simulink model "proc_control_node"  (R2021b)
settings: Solver=FixedStepAuto  StartTime=0.0  StopTime=inf  FixedStep=simulink.sampletime  RelTol=1e-3
model workspace (MAT data in the model file):
  SL_ROS_VariableLengthArrays_MaxSizes.CommonInfo.ArrayTruncateAction = 'EmitWarning'
  SL_ROS_VariableLengthArrays_MaxSizes.MsgTypeMap = containers.Map
  SL_ROS_VariableLengthArrays_MaxSizes.MsgTypeMap.serialization.keys = {'trajectory_msgs/MultiDOFJointTrajectoryPoint'}
  SL_ROS_VariableLengthArrays_MaxSizes.MsgTypeMap.serialization.values{1}(1).PropertyName = 'Accelerations'
  SL_ROS_VariableLengthArrays_MaxSizes.MsgTypeMap.serialization.values{1}(1).DataType = 'geometry_msgs/Twist'
  SL_ROS_VariableLengthArrays_MaxSizes.MsgTypeMap.serialization.values{1}(1).MaxLength = 6000
  SL_ROS_VariableLengthArrays_MaxSizes.MsgTypeMap.serialization.values{1}(2).PropertyName = 'Transforms'
  SL_ROS_VariableLengthArrays_MaxSizes.MsgTypeMap.serialization.values{1}(2).DataType = 'geometry_msgs/Transform'
  SL_ROS_VariableLengthArrays_MaxSizes.MsgTypeMap.serialization.values{1}(2).MaxLength = 6000
  SL_ROS_VariableLengthArrays_MaxSizes.MsgTypeMap.serialization.values{1}(3).PropertyName = 'Velocities'
  SL_ROS_VariableLengthArrays_MaxSizes.MsgTypeMap.serialization.values{1}(3).DataType = 'geometry_msgs/Twist'
  SL_ROS_VariableLengthArrays_MaxSizes.MsgTypeMap.serialization.values{1}(3).MaxLength = 6000
  SL_ROS_VariableLengthArrays_MaxSizes.MsgTypeMap.serialization.uniformity = 0
  SL_ROS_VariableLengthArrays_MaxSizes.MsgTypeMap.serialization.keyType = 'char'
  SL_ROS_VariableLengthArrays_MaxSizes.MsgTypeMap.serialization.valueType = 'any'
undefined symbols (not defined in the file or in its folder): InitAUVPlant, InitController, MPC, physics, simulation, simulink
libraries: robotlib x36, aerolibutil x7, sharedtransform x5, simulink_extras x3
settings Model: SimulationMode=accelerator  PacingRate=1.400000  Creator=lamarre  LastModifiedBy=lamarre
settings OptimizationCC: StrengthReduction=on  PassReuseOutputArgsAs=Individual arguments  ZeroExternalMemoryAtStartup=off  ZeroInternalMemoryAtStartup=off  EfficientFloat2IntCast=on  LifeSpan=inf  MaxStackSize=64  OptimizeBlockOrder=speed  OptimizationPriority=Speed  MultiThreadedLoops=on  EfficientTunableParamExpr=on
settings DebuggingCC: ReadBeforeWriteMsg=DisableAll  WriteAfterWriteMsg=DisableAll  WriteAfterReadMsg=DisableAll  MultiTaskDSMMsg=none  ParameterTunabilityLossMsg=error  UnderSpecifiedDimensionMsg=warning
settings HardwareCC: ProdLargestAtomicInteger=Long  ProdLargestAtomicFloat=Double  ProdLongLongMode=on  ProdHWDeviceType=ARM Compatible->ARM 64-bit (LLP64)
settings ModelReferenceCC: UpdateModelReferenceTargets=IfOutOfDate
settings SFSimCC: SFSimEcho=off  MATLABDynamicMemAlloc=off  SimTargetLang=C++
settings RTWCC: Description=Embedded Coder  SystemTargetFile=ert.tlc  HardwareBoard=Robot Operating System (ROS)  TLCOptions="-aInlineSetEventsForThisBaseRateFcn=TLC_FALSE -aSuppressMultiTaskScheduler=TLC_FALSE  -aRateBasedStepFcn=0"  GenCodeOnly=on  TemplateMakefile=ert_default_tmf  Toolchain=Catkin  BuildConfiguration=Faster Runs  TargetLang=C++
settings CodeAppCC: ForceParamTrailComments=on  IgnoreCustomStorageClasses=off  IgnoreTestpoints=on  OperatorAnnotations=on  SimulinkDataObjDesc=on  SFDataObjDesc=on  InsertBlockDesc=on
settings ERTTargetCC: TargetLangStandard=C++11 (ISO)  CodeInterfacePackaging=C++ class  SupportContinuousTime=on  SupportVariableSizeSignals=on  ExtModeMexArgs='192.168.0.31' 0 17725  RootIOFormat=Structure reference

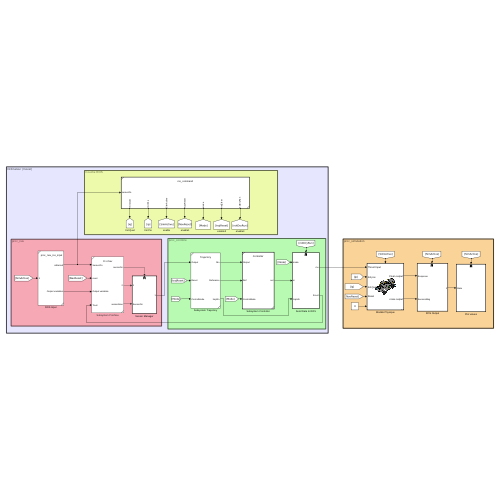
[thumbnail: Simulink's stored preview of the top-level diagram]
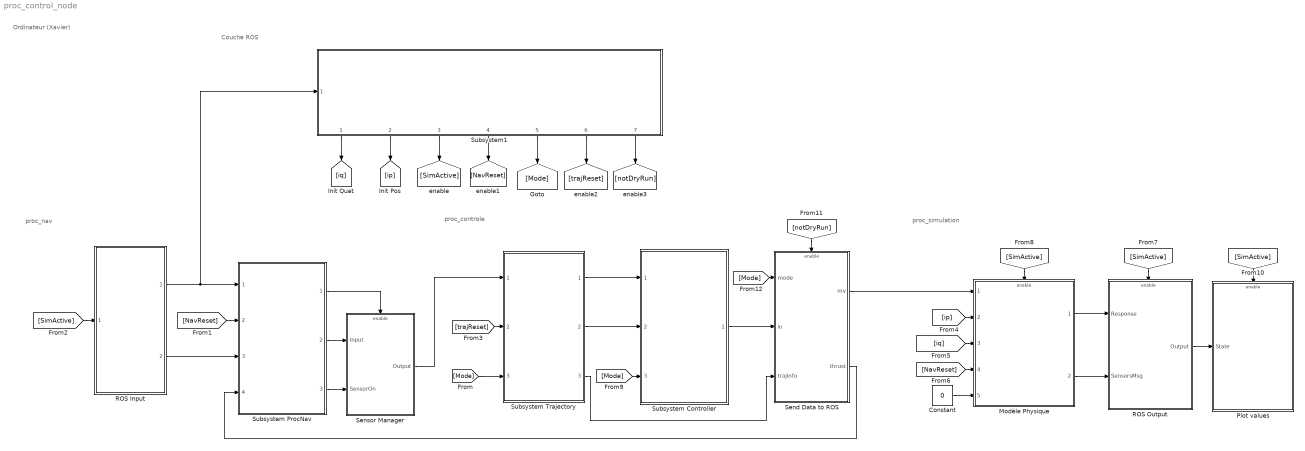
== system proc_control_node ==
  note: proc_simulation
  note: proc_nav
  note: Couche ROS
  note: Ordinateur (Xavier)
  note: proc_controle
  Constant : Constant  Value=0
  Modèle Physique : Subsystem  InitFcn=InitAUVPlant;  ReferencedSubsystem=AUVPlant
  Plot values : Subsystem
  ROS Input : Subsystem  SystemSampleTime=simulink.procNav.sampletime  ReferencedSubsystem=proc_nav_ros_input
  ROS Output : Subsystem
  Send Data to ROS : Subsystem  SystemSampleTime=1/10
  Sensor Manager : Subsystem
  Subsystem Controller : Subsystem  InitFcn=InitController;  StopFcn=|  TreatAsAtomicUnit=on  SystemSampleTime=1/10  ReferencedSubsystem=Controller
      | %rosinit;
      | %[pub,msg] = rospublisher("/provider_thruster/thruster_pwm","std_msgs/UInt16MultiArray");
      | 
      | %msg.Data = [1500,1500,1500,1500,1500,1500,1500,1500];
      | 
      | %send(pub,msg);
      | %rosshutdown
  Subsystem ProcNav : Subsystem  SystemSampleTime=simulink.procNav.sampletime  ReferencedSubsystem=ProcNav
      settings: MinAlgLoopOccurrences=on
  Subsystem Trajectory : Subsystem  InitFcn=|  ReferencedSubsystem=Trajectory
      | InitTrajectory
      | %trajec;
  Subsystem1 : Subsystem  TreatAsAtomicUnit=on  SystemSampleTime=1/10  ReferencedSubsystem=ros_command
      settings: PortSchema="{\"entries\":[{\"content\":{\"sides\":[{\"content\":{\"connectorIds\":[\"In1\"]},\"type\":\"ConnectorPlacement.EquallySpacedRectSide\",\"uuid\":\"274bdad9-d78d-43c8-9ae1-3ca28a37e384\"},{\"content\":{\"connectorIds\":[],\"side\":\"RIGHT\"},\"type\":\"ConnectorPlacement.EquallySpacedRectSide\",\"uuid\":\"7ee2482a-029c-4d86-ab0a-df49e4223d0b\"},{\"content\":{\"connectorIds\":[],\"side\":\"TOP\"},\"type\":\"ConnectorPlacement.EquallySpacedRectSide\",\"uuid\":\"c10c93c4-dac3-4bbe-8faf-09a38e374d51\"},{\"content\":{\"connectorIds\":[\"Out1\",\"Out2\",\"Out3\",\"Out4\",\"Out5\",\"Out6\",\"Out7\"],\"side\":\"BOTTOM\"},\"type\":\"ConnectorPlacement.EquallySpacedRectSide\",\"uuid\":\"2cd10030-3eb5-48df-9d04-da9a86e3b973\"}]},\"type\":\"ConnectorPlacement.EquallySpacedConnector\",\"uuid\":\"6c3543f2-9cdd-4b68-a1ea-0df50348da33\"}],\"packageUris\":[\"http://schema.mathworks.com/mf0/Connector/R2020b\"],\"version\":\"1.0\"}"
  wires:
  Subsystem1/5 -> [Mode]
  [NavReset] -> Subsystem ProcNav/2
  Send Data to ROS/1(mv) -> Modèle Physique/1
  Modèle Physique/1 -> ROS Output/1(Response)
  [SimActive] -> Modèle Physique/Enable
  Subsystem1/3 -> [SimActive]
  [trajReset] -> Subsystem Trajectory/2
  [NavReset] -> Modèle Physique/4
  [ip] -> Modèle Physique/2
  [SimActive] -> Plot values/Enable
  Subsystem1/1 -> [iq]
  [SimActive] -> ROS Output/Enable
  Subsystem1/2 -> [ip]
  Subsystem1/4 -> [NavReset]
  Sensor Manager/1(Output) -> Subsystem Trajectory/1
  Modèle Physique/2 -> ROS Output/2(SensorsMsg)
  Subsystem Trajectory/3 -> Send Data to ROS/3(trajInfo)
  Subsystem Controller/1 -> Send Data to ROS/2(in)
  ROS Output/1(Output) -> Plot values/1(State)
  [Mode] -> Subsystem Trajectory/3
  [iq] -> Modèle Physique/3
  Subsystem ProcNav/2 -> Sensor Manager/1(Input)
  Subsystem ProcNav/3 -> Sensor Manager/2(SensorOn)
  [SimActive] -> ROS Input/1
  Subsystem1/6 -> [trajReset]
  Subsystem ProcNav/1 -> Sensor Manager/Enable
  ROS Input/1 -> Subsystem1/1, Subsystem ProcNav/1
  ROS Input/2 -> Subsystem ProcNav/3
  Subsystem1/7 -> [notDryRun]
  [notDryRun] -> Send Data to ROS/Enable
  Subsystem Trajectory/1 -> Subsystem Controller/1
  Subsystem Trajectory/2 -> Subsystem Controller/2
  [Mode] -> Subsystem Controller/3
  Send Data to ROS/2(thrust) -> Subsystem ProcNav/4
  [Mode] -> Send Data to ROS/1(mode)
  Constant/1 -> Modèle Physique/5

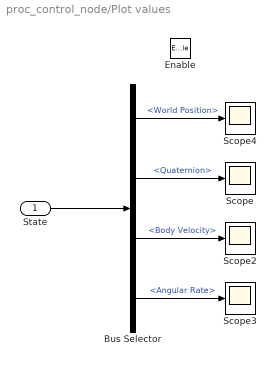
== system proc_control_node/Plot values ==
  State : Inport
  Enable : EnablePort
  Bus Selector : BusSelector  OutputSignals=signal1.World Position,signal1.Quaternion,signal2.Body Velocity,signal2.Angular Rate
  Scope{,2..4} (4 alike) : Scope
  wires:
  Bus Selector/4 -> Scope3/1  "<Angular Rate>"
  State/1 -> Bus Selector/1
  Bus Selector/2 -> Scope/1  "<Quaternion>"
  Bus Selector/3 -> Scope2/1  "<Body Velocity>"
  Bus Selector/1 -> Scope4/1  "<World Position>"

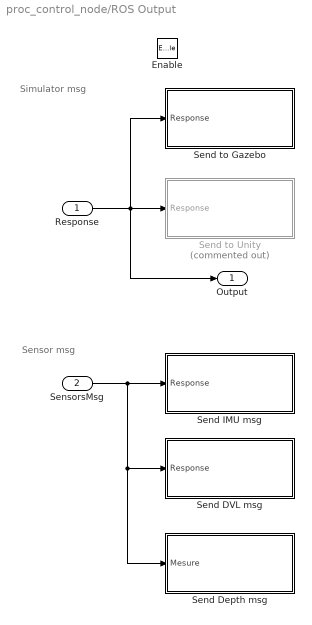
== system proc_control_node/ROS Output ==
  note: Sensor msg
  note: Simulator msg
  Response : Inport
  SensorsMsg : Inport  Port=2
  Enable : EnablePort
  Send DVL msg : Subsystem
  Send Depth msg : Subsystem
  Send IMU msg : Subsystem
  Send to Gazebo : Subsystem  InitFcn=""
  Send to Unity : Subsystem  Commented=on
  Output : Outport
  wires:
  Response/1 -> Send to Unity/1(Response), Output/1, Send to Gazebo/1(Response)
  SensorsMsg/1 -> Send Depth msg/1(Mesure), Send DVL msg/1(Response), Send IMU msg/1(Response)

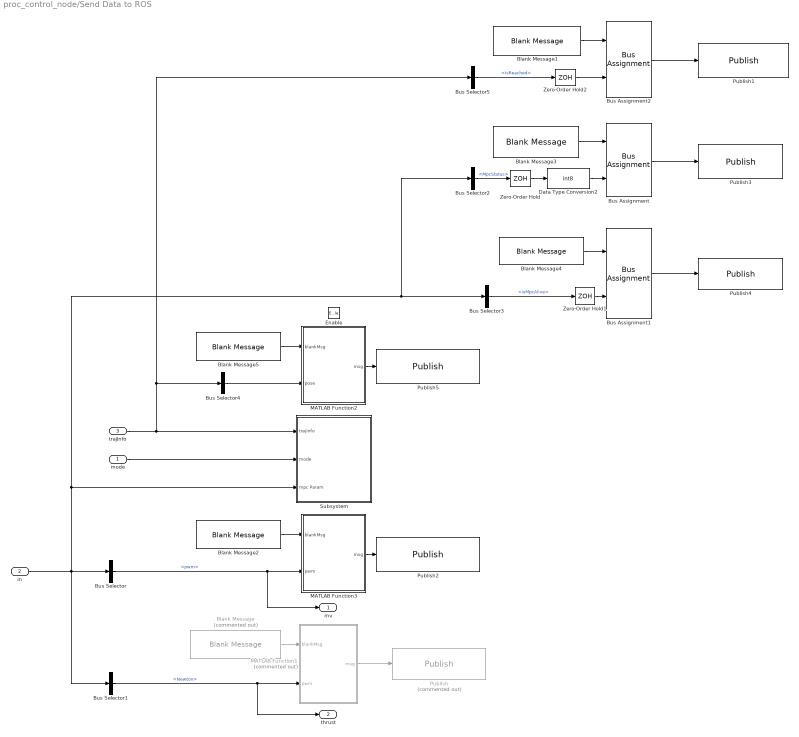
== system proc_control_node/Send Data to ROS ==
  mode : Inport
  in : Inport  Port=2
  trajInfo : Inport  Port=3
  Enable : EnablePort
  Blank Message : robotlib/Blank Message  Commented=on  messageClass=Message  entityType=std_msgs/Int8MultiArray  messageType=std_msgs/Int8MultiArray  SampleTime=inf  legacyBusStruct=off
  Blank Message1 : robotlib/Blank Message  messageClass=Message  entityType=std_msgs/Bool  messageType=std_msgs/Bool  SampleTime=1  legacyBusStruct=off
  Blank Message2 : robotlib/Blank Message  messageClass=Message  entityType=std_msgs/UInt16MultiArray  messageType=std_msgs/UInt16MultiArray  SampleTime=inf  legacyBusStruct=off
  Blank Message3 : robotlib/Blank Message  messageClass=Message  entityType=std_msgs/Int8  messageType=std_msgs/Int8  SampleTime=1  legacyBusStruct=off
  Blank Message4 : robotlib/Blank Message  messageClass=Message  entityType=std_msgs/Bool  messageType=std_msgs/Bool  SampleTime=1  legacyBusStruct=off
  Blank Message5 : robotlib/Blank Message  messageClass=Message  entityType=geometry_msgs/Pose  messageType=geometry_msgs/Pose  SampleTime=inf  legacyBusStruct=off
  Bus Assignment : BusAssignment  AssignedSignals=Data
  Bus Assignment1 : BusAssignment  AssignedSignals=Data
  Bus Assignment2 : BusAssignment  AssignedSignals=Data
  Bus Selector : BusSelector  OutputSignals=pwm
  Bus Selector1 : BusSelector  OutputSignals=Newton
  Bus Selector2 : BusSelector  OutputSignals=MpcStatus
  Bus Selector3 : BusSelector  OutputSignals=isMpcAlive
  Bus Selector4 : BusSelector  OutputSignals=initWpt  OutputAsBus=on
  Bus Selector5 : BusSelector  OutputSignals=isReached
  Data Type Conversion2 : DataTypeConversion  OutDataTypeStr=int8  RndMeth=Nearest
  MATLAB Function1 : MATLAB Function  Commented=on  TreatAsAtomicUnit=on  SystemSampleTime=MPC.Ts
  MATLAB Function2 : MATLAB Function  TreatAsAtomicUnit=on  SystemSampleTime=MPC.Ts
  MATLAB Function3 : MATLAB Function  TreatAsAtomicUnit=on  SystemSampleTime=MPC.Ts
  Publish : robotlib/Publish  Commented=on  topicSource=Specify your own  topic=/telemetry/thruster_newton  messageType=std_msgs/Int8MultiArray  legacyBusStruct=off  messageQueueLength=1
  Publish1 : robotlib/Publish  topicSource=Specify your own  topic=proc_control/target_reached  messageType=std_msgs/Bool  legacyBusStruct=off  messageQueueLength=1
  Publish2 : robotlib/Publish  topicSource=Specify your own  topic=/provider_thruster/thruster_pwm  messageType=std_msgs/UInt16MultiArray  legacyBusStruct=off  messageQueueLength=1
  Publish3 : robotlib/Publish  topicSource=Specify your own  topic=proc_control/mpc_status  messageType=std_msgs/Int8  legacyBusStruct=off  messageQueueLength=1
  Publish4 : robotlib/Publish  topicSource=Specify your own  topic=proc_control/is_mpc_active  messageType=std_msgs/Bool  legacyBusStruct=off  messageQueueLength=1
  Publish5 : robotlib/Publish  topicSource=Select from ROS network  topic=/proc_planner/initial_pose  messageType=geometry_msgs/Pose  legacyBusStruct=off  messageQueueLength=1
  Subsystem : Subsystem  TreatAsAtomicUnit=on  SystemSampleTime=1
  Zero-Order Hold : ZeroOrderHold
  Zero-Order Hold1 : ZeroOrderHold
  Zero-Order Hold2 : ZeroOrderHold
  mv : Outport
  thrust : Outport  Port=2
  wires:
  MATLAB Function1/1(msg) -> Publish/1
  Blank Message/1 -> MATLAB Function1/1(blankMsg)
  Bus Selector1/1 -> thrust/1, MATLAB Function1/2(pwm)  "<Newton>"
  MATLAB Function3/1(msg) -> Publish2/1
  Blank Message2/1 -> MATLAB Function3/1(blankMsg)
  Blank Message3/1 -> Bus Assignment/1
  Bus Assignment/1 -> Publish3/1
  Data Type Conversion2/1 -> Bus Assignment/2
  Bus Selector2/1 -> Zero-Order Hold/1  "<MpcStatus>"
  Bus Selector3/1 -> Zero-Order Hold1/1  "<isMpcAlive>"
  Bus Assignment1/1 -> Publish4/1
  Blank Message4/1 -> Bus Assignment1/1
  Zero-Order Hold/1 -> Data Type Conversion2/1
  Blank Message1/1 -> Bus Assignment2/1
  Bus Assignment2/1 -> Publish1/1
  Zero-Order Hold2/1 -> Bus Assignment2/2
  Zero-Order Hold1/1 -> Bus Assignment1/2
  Bus Selector/1 -> mv/1, MATLAB Function3/2(pwm)  "<pwm>"
  in/1 -> Subsystem/3(mpc Param), Bus Selector2/1, Bus Selector3/1, Bus Selector1/1, Bus Selector/1
  mode/1 -> Subsystem/2(mode)
  trajInfo/1 -> Bus Selector5/1, Bus Selector4/1, Subsystem/1(trajInfo)
  MATLAB Function2/1(msg) -> Publish5/1
  Blank Message5/1 -> MATLAB Function2/1(blankMsg)
  Bus Selector4/1 -> MATLAB Function2/2(pose)
  Bus Selector5/1 -> Zero-Order Hold2/1  "<isReached>"

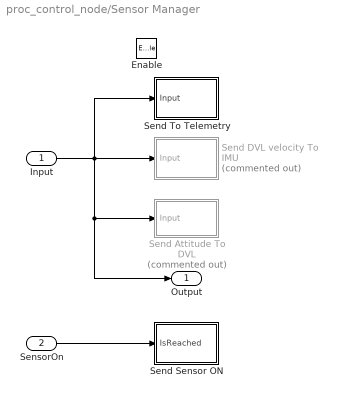
== system proc_control_node/Sensor Manager ==
  Input : Inport
  SensorOn : Inport  Port=2
  Enable : EnablePort
  Send Attitude To DVL : Subsystem  Commented=on
  Send DVL velocity To IMU : Subsystem  Commented=on
  Send Sensor ON : Subsystem
  "Send To Telemetry " : Subsystem
  Output : Outport
  wires:
  Input/1 -> Send DVL velocity To IMU/1(Input), Output/1, Send Attitude To DVL/1(Input), "Send To Telemetry "/1(Input)
  SensorOn/1 -> Send Sensor ON/1(IsReached)

== system proc_control_node/ROS Output/Send DVL msg ==
  Response : Inport
  "   " : robotlib/Blank Message  messageClass=Message  entityType=sonia_common/BodyVelocityDVL  messageType=sonia_common/BodyVelocityDVL  SampleTime=simulation.sensors.dvl.sampletime  legacyBusStruct=off
  Bus Selector : BusSelector  OutputSignals=DVL Velocity
  MATLAB Function : MATLAB Function  TreatAsAtomicUnit=on  SystemSampleTime=simulation.sensors.dvl.sampletime
  Publish : robotlib/Publish  topicSource=Specify your own  topic=/proc_simulation/dvl_velocity  messageType=sonia_common/BodyVelocityDVL  legacyBusStruct=off  messageQueueLength=1
      link override SinkBlock: ROSTopic=/gazebo/set_model_state  ROSMessageType=gazebo_msgs/ModelState  SLBusName=SL_Bus_plant_gazebo_msgs_ModelState  ModelName=plant  BlockId=Pub_plant_206
  wires:
  Bus Selector/1 -> MATLAB Function/2(bodyVelocity)  "<DVL Velocity>"
  "   "/1 -> MATLAB Function/1(blankMsg)
  MATLAB Function/1(msg) -> Publish/1
  Response/1 -> Bus Selector/1

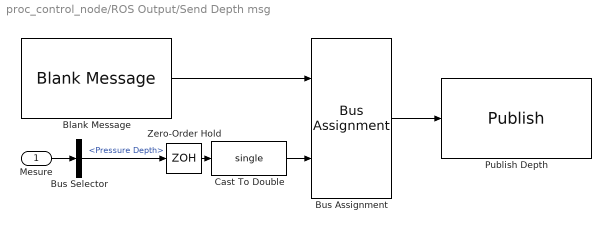
== system proc_control_node/ROS Output/Send Depth msg ==
  Mesure : Inport
  Blank Message : robotlib/Blank Message  messageClass=Message  entityType=std_msgs/Float32  messageType=std_msgs/Float32  SampleTime=simulation.sensors.depth.sampletime  legacyBusStruct=off
  Bus Assignment : BusAssignment  AssignedSignals=Data
  Bus Selector : BusSelector  OutputSignals=Pressure Depth
  Cast To Double : DataTypeConversion  OutDataTypeStr=single
  Publish Depth : robotlib/Publish  topicSource=Specify your own  topic=/proc_simulation/depth  messageType=std_msgs/Float32  legacyBusStruct=off  messageQueueLength=1
  Zero-Order Hold : ZeroOrderHold  SampleTime=simulation.sensors.depth.sampletime
  wires:
  Mesure/1 -> Bus Selector/1
  Bus Assignment/1 -> Publish Depth/1
  Blank Message/1 -> Bus Assignment/1
  Cast To Double/1 -> Bus Assignment/2
  Bus Selector/1 -> Zero-Order Hold/1  "<Pressure Depth>"
  Zero-Order Hold/1 -> Cast To Double/1

== system proc_control_node/ROS Output/Send IMU msg ==
  note: cvt 3840 2160 60
  Response : Inport
  "   " : robotlib/Blank Message  messageClass=Message  entityType=sensor_msgs/Imu  messageType=sensor_msgs/Imu  SampleTime=simulation.sensors.imu.sampletime  legacyBusStruct=off
  Bus Selector : BusSelector  OutputSignals=Angular Rate,Quaternion,Linear Acceleration
  MATLAB Function : MATLAB Function  TreatAsAtomicUnit=on  SystemSampleTime=simulation.sensors.imu.sampletime
  Publish imu_info : robotlib/Publish  topicSource=Specify your own  topic=/proc_simulation/imu_info  messageType=sensor_msgs/Imu  legacyBusStruct=off  messageQueueLength=1
      link override SinkBlock: ROSTopic=/gazebo/set_model_state  ROSMessageType=gazebo_msgs/ModelState  SLBusName=SL_Bus_plant_gazebo_msgs_ModelState  ModelName=plant  BlockId=Pub_plant_206
  wires:
  Bus Selector/1 -> MATLAB Function/2(angularRate)  "<Angular Rate>"
  "   "/1 -> MATLAB Function/1(blankMsg)
  MATLAB Function/1(msg) -> Publish imu_info/1
  Response/1 -> Bus Selector/1
  Bus Selector/2 -> MATLAB Function/3(quaternion)  "<Quaternion>"
  Bus Selector/3 -> MATLAB Function/4(linearAcc)  "<Linear Acceleration>"

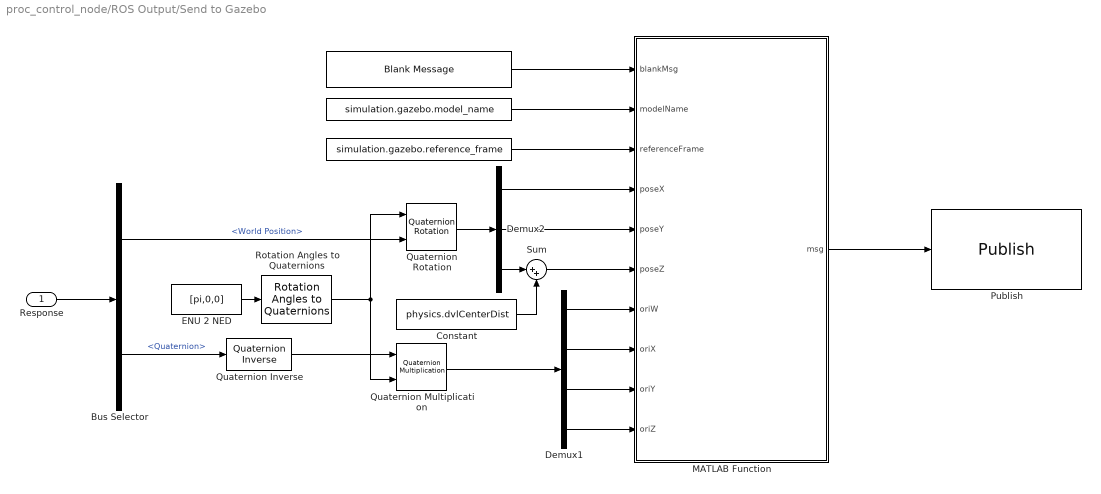
== system proc_control_node/ROS Output/Send to Gazebo ==
  Response : Inport
  " " : Constant  Value=simulation.gazebo.model_name  VectorParams1D=off
  "  " : Constant  Value=simulation.gazebo.reference_frame
  "   " : robotlib/Blank Message  messageClass=Message  entityType=gazebo_msgs/ModelState  messageType=gazebo_msgs/ModelState  SampleTime=simulation.gazebo.sampletime  legacyBusStruct=off
  Bus Selector : BusSelector  OutputSignals=signal1.World Position,signal1.Quaternion
  Constant : Constant  Value=physics.dvlCenterDist
  Demux1 : Demux
  Demux2 : Demux  Outputs=3
  ENU 2 NED : Constant  Value=[pi,0,0]
  MATLAB Function : MATLAB Function  TreatAsAtomicUnit=on  SystemSampleTime=simulation.gazebo.sampletime
  Publish : robotlib/Publish  topicSource=Select from ROS network  topic=/gazebo/set_model_state  messageType=gazebo_msgs/ModelState  legacyBusStruct=off  messageQueueLength=1
      link override SinkBlock: ROSTopic=/gazebo/set_model_state  ROSMessageType=gazebo_msgs/ModelState  SLBusName=SL_Bus_plant_gazebo_msgs_ModelState  ModelName=plant  BlockId=Pub_plant_206
  Quaternion Inverse : aerolibutil/Quaternion Inverse
  Quaternion Multiplication : aerolibutil/Quaternion Multiplication
  Quaternion Rotation : aerolibutil/Quaternion Rotation
  Rotation Angles to Quaternions : sharedtransform/Rotation Angles to Quaternions  rotationOrder=XYZ  aMode=aMode
      settings: SourceProductBaseCode=AE,PW,DR,MT,UV,VE
  Sum : Sum  Inputs=|++
  wires:
  "   "/1 -> MATLAB Function/1(blankMsg)
  "  "/1 -> MATLAB Function/3(referenceFrame)
  " "/1 -> MATLAB Function/2(modelName)
  Demux1/1 -> MATLAB Function/7(oriW)
  Demux1/2 -> MATLAB Function/8(oriX)
  Demux1/3 -> MATLAB Function/9(oriY)
  Demux1/4 -> MATLAB Function/10(oriZ)
  MATLAB Function/1(msg) -> Publish/1
  Response/1 -> Bus Selector/1
  Sum/1 -> MATLAB Function/6(poseZ)
  Constant/1 -> Sum/2
  Bus Selector/2 -> Quaternion Inverse/1  "<Quaternion>"
  ENU 2 NED/1 -> Rotation Angles to Quaternions/1
  Rotation Angles to Quaternions/1 -> Quaternion Multiplication/2, Quaternion Rotation/1
  Bus Selector/1 -> Quaternion Rotation/2  "<World Position>"
  Demux2/3 -> Sum/1
  Demux2/2 -> MATLAB Function/5(poseY)
  Demux2/1 -> MATLAB Function/4(poseX)
  Quaternion Rotation/1 -> Demux2/1
  Quaternion Multiplication/1 -> Demux1/1
  Quaternion Inverse/1 -> Quaternion Multiplication/1

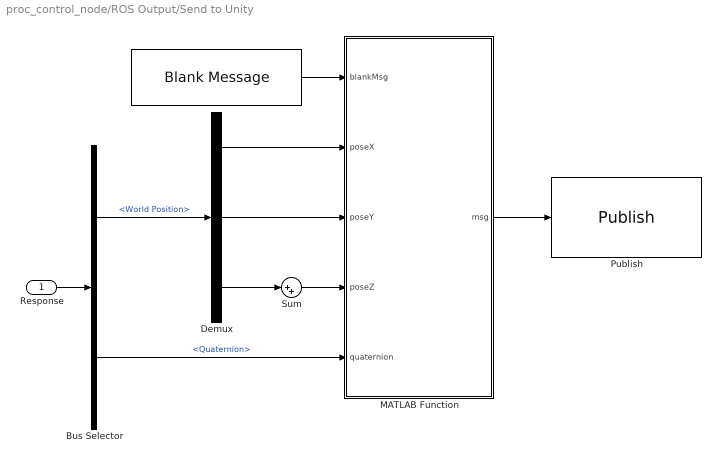
== system proc_control_node/ROS Output/Send to Unity ==
  Response : Inport
  "   " : robotlib/Blank Message  messageClass=Message  entityType=geometry_msgs/Pose  messageType=geometry_msgs/Pose  SampleTime=simulation.unity.sampletime  legacyBusStruct=off
  Bus Selector : BusSelector  OutputSignals=signal1.World Position,signal1.Quaternion
  Demux : Demux  Outputs=3
  MATLAB Function : MATLAB Function  TreatAsAtomicUnit=on  SystemSampleTime=simulation.unity.sampletime
  Publish : robotlib/Publish  topicSource=Specify your own  topic=/pos_rot  messageType=geometry_msgs/Pose  legacyBusStruct=off  messageQueueLength=1
      link override SinkBlock: ROSTopic=/gazebo/set_model_state  ROSMessageType=gazebo_msgs/ModelState  SLBusName=SL_Bus_plant_gazebo_msgs_ModelState  ModelName=plant  BlockId=Pub_plant_206
  Sum : Sum  Inputs=|++
  wires:
  Bus Selector/1 -> Demux/1  "<World Position>"
  "   "/1 -> MATLAB Function/1(blankMsg)
  MATLAB Function/1(msg) -> Publish/1
  Response/1 -> Bus Selector/1
  Sum/1 -> MATLAB Function/4(poseZ)
  Demux/1 -> MATLAB Function/2(poseX)
  Demux/2 -> MATLAB Function/3(poseY)
  Demux/3 -> Sum/1
  Bus Selector/2 -> MATLAB Function/5(quaternion)  "<Quaternion>"

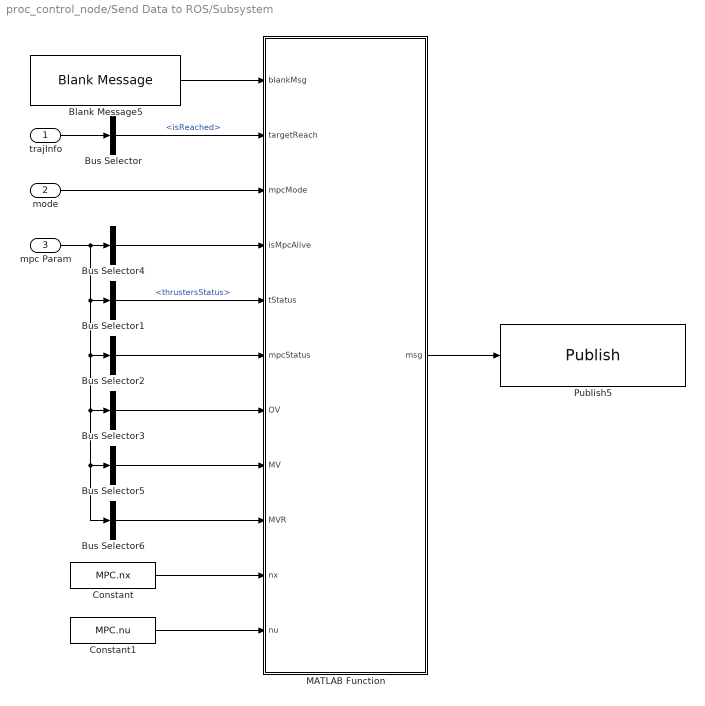
== system proc_control_node/Send Data to ROS/Subsystem ==
  trajInfo : Inport
  mode : Inport  Port=2
  mpc Param : Inport  Port=3
  Blank Message5 : robotlib/Blank Message  messageClass=Message  entityType=sonia_common/MpcInfo  messageType=sonia_common/MpcInfo  SampleTime=1  legacyBusStruct=off
  Bus Selector : BusSelector  OutputSignals=isReached
  Bus Selector1 : BusSelector  OutputSignals=mpcParam.thrustersStatus
  Bus Selector2 : BusSelector  OutputSignals=MpcStatus  OutputAsBus=on
  Bus Selector3 : BusSelector  OutputSignals=mpcParam.ywt  OutputAsBus=on
  Bus Selector4 : BusSelector  OutputSignals=isMpcAlive  OutputAsBus=on
  Bus Selector5 : BusSelector  OutputSignals=mpcParam.mvwt  OutputAsBus=on
  Bus Selector6 : BusSelector  OutputSignals=mpcParam.dmwwt  OutputAsBus=on
  Constant : Constant  Value=MPC.nx
  Constant1 : Constant  Value=MPC.nu
  MATLAB Function : MATLAB Function  TreatAsAtomicUnit=on  SystemSampleTime=1
  Publish5 : robotlib/Publish  topicSource=Specify your own  topic=proc_control/controller_info  messageType=sonia_common/MpcInfo  legacyBusStruct=off  messageQueueLength=1
  wires:
  MATLAB Function/1(msg) -> Publish5/1
  Blank Message5/1 -> MATLAB Function/1(blankMsg)
  Bus Selector1/1 -> MATLAB Function/5(tStatus)  "<thrustersStatus>"
  Bus Selector2/1 -> MATLAB Function/6(mpcStatus)
  Bus Selector3/1 -> MATLAB Function/7(OV)
  Bus Selector5/1 -> MATLAB Function/8(MV)
  mpc Param/1 -> Bus Selector2/1, Bus Selector3/1, Bus Selector6/1, Bus Selector5/1, Bus Selector1/1, Bus Selector4/1
  Bus Selector6/1 -> MATLAB Function/9(MVR)
  Constant/1 -> MATLAB Function/10(nx)
  Constant1/1 -> MATLAB Function/11(nu)
  Bus Selector4/1 -> MATLAB Function/4(isMpcAlive)
  mode/1 -> MATLAB Function/3(mpcMode)
  trajInfo/1 -> Bus Selector/1
  Bus Selector/1 -> MATLAB Function/2(targetReach)  "<isReached>"

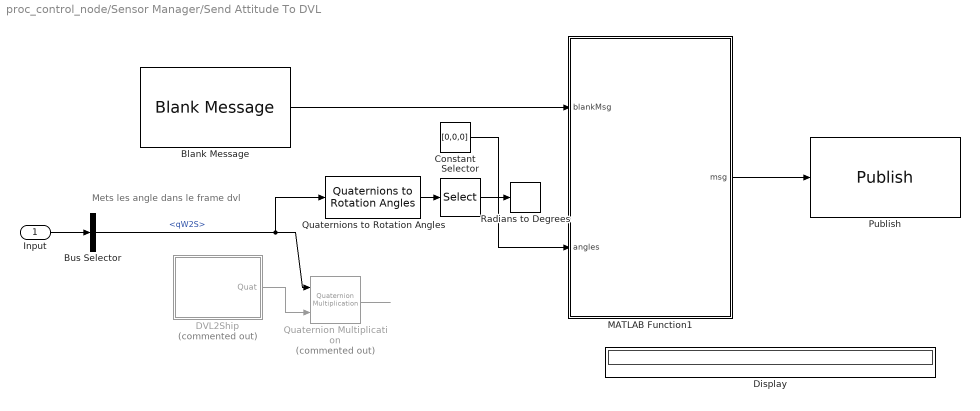
== system proc_control_node/Sensor Manager/Send Attitude To DVL ==
  note: Mets les angle dans le frame dvl
  Input : Inport
  Blank Message : robotlib/Blank Message  messageClass=Message  entityType=geometry_msgs/Vector3  messageType=geometry_msgs/Vector3  SampleTime=-1  legacyBusStruct=off
  Bus Selector : BusSelector  OutputSignals=qW2S
  Constant : Constant  Value=[0,0,0]
  DVL2Ship : Subsystem  Commented=on
  Display : Display
  MATLAB Function1 : MATLAB Function  TreatAsAtomicUnit=on  SystemSampleTime=1
  Publish : robotlib/Publish  topicSource=Select from ROS network  topic=/provider_dvl/set_angles  messageType=geometry_msgs/Vector3  legacyBusStruct=off  messageQueueLength=1
  Quaternion Multiplication : aerolibutil/Quaternion Multiplication  Commented=on
  Quaternions to Rotation Angles : sharedtransform/Quaternions to Rotation Angles  rotationOrder=ZYX  aMode=aMode
      settings: SourceProductBaseCode=AE,PW,DR,MT,UV,VE
  Radians to Degrees : simulink_extras/Transformations/Radians to Degrees
  Selector : Selector  InputPortWidth=3  IndexOptions=Index vector (dialog)  Indices=[3,2,1]  OutputSizes=1
  wires:
  Blank Message/1 -> MATLAB Function1/1(blankMsg)
  MATLAB Function1/1(msg) -> Publish/1
  Input/1 -> Bus Selector/1
  Bus Selector/1 -> Quaternions to Rotation Angles/1, Quaternion Multiplication/1  "<qW2S>"
  Quaternion Multiplication/1 -> ?
  DVL2Ship/1(Quat) -> Quaternion Multiplication/2
  Quaternions to Rotation Angles/1 -> Selector/1
  Selector/1 -> Radians to Degrees/1
  Constant/1 -> MATLAB Function1/2(angles)

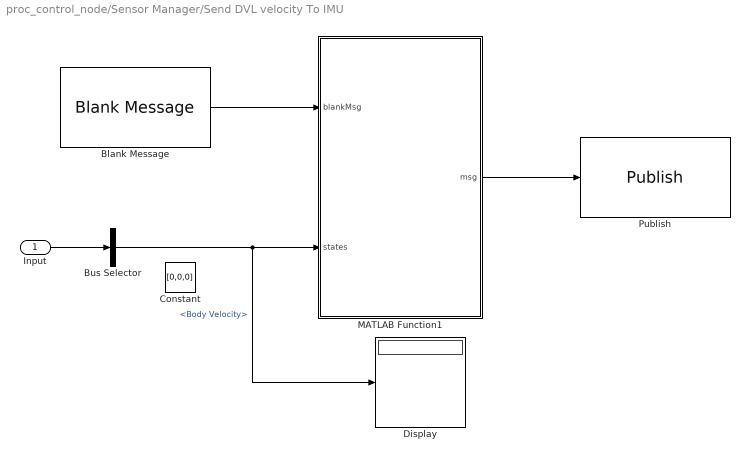
== system proc_control_node/Sensor Manager/Send DVL velocity To IMU ==
  Input : Inport
  Blank Message : robotlib/Blank Message  messageClass=Message  entityType=geometry_msgs/Twist  messageType=geometry_msgs/Twist  SampleTime=inf  legacyBusStruct=off
  Bus Selector : BusSelector  OutputSignals=Body Velocity
  Constant : Constant  Value=[0,0,0]
  Display : Display
  MATLAB Function1 : MATLAB Function  TreatAsAtomicUnit=on  SystemSampleTime=1/20
  Publish : robotlib/Publish  topicSource=Select from ROS network  topic=/proc_nav/dvl_velocity  messageType=geometry_msgs/Twist  legacyBusStruct=off  messageQueueLength=1
  wires:
  Blank Message/1 -> MATLAB Function1/1(blankMsg)
  MATLAB Function1/1(msg) -> Publish/1
  Input/1 -> Bus Selector/1
  Bus Selector/1 -> Display/1, MATLAB Function1/2(states)  "<Body Velocity>"

== system proc_control_node/Sensor Manager/Send Sensor ON ==
  IsReached : Inport
  Blank Message : robotlib/Blank Message  messageClass=Message  entityType=std_msgs/Bool  messageType=std_msgs/Bool  SampleTime=-1  legacyBusStruct=off
  Bus Assignment : BusAssignment  AssignedSignals=Data
  Cast To Boolean : DataTypeConversion  OutDataTypeStr=boolean
  Publish : robotlib/Publish  topicSource=Specify your own  topic=proc_control/sensor_on  messageType=std_msgs/Bool  legacyBusStruct=off  messageQueueLength=1
  Zero-Order Hold : ZeroOrderHold
  wires:
  Blank Message/1 -> Bus Assignment/1
  IsReached/1 -> Cast To Boolean/1
  Bus Assignment/1 -> Zero-Order Hold/1
  Cast To Boolean/1 -> Bus Assignment/2
  Zero-Order Hold/1 -> Publish/1

== system proc_control_node/Sensor Manager/Send To Telemetry  ==
  Input : Inport
  Blank Message : robotlib/Blank Message  messageClass=Message  entityType=nav_msgs/Odometry  messageType=nav_msgs/Odometry  SampleTime=inf  legacyBusStruct=off
  Conversion d'unité : Subsystem
  MATLAB Function1 : MATLAB Function  TreatAsAtomicUnit=on  SystemSampleTime=simulink.procNav.sampletime
  Publish : robotlib/Publish  topicSource=Specify your own  topic=/telemetry/auv_states/  messageType=nav_msgs/Odometry  legacyBusStruct=off  messageQueueLength=1
  Send to Gazebo : Subsystem  Commented=on  InitFcn=""
  Send to Unity : Subsystem  Commented=on
  wires:
  Blank Message/1 -> MATLAB Function1/1(blankMsg)
  MATLAB Function1/1(msg) -> Publish/1
  Input/1 -> Send to Unity/1(Response), Send to Gazebo/1(Response), Conversion d'unité/1(In1)
  Conversion d'unité/1(states) -> MATLAB Function1/2(states)

== system proc_control_node/Sensor Manager/Send Attitude To DVL/DVL2Ship ==
  Constant6 : Constant  Value=0
  Delay : Delay  DelayLength=1  InitialCondition=1
  Subsystem2 : Subsystem
  Quat : Outport
  wires:
  Subsystem2/1(Quat) -> Quat/1
  Constant6/1 -> Delay/1
  Delay/1 -> Subsystem2/Enable

== system proc_control_node/Sensor Manager/Send To Telemetry /Conversion d'unité ==
  In1 : Inport
  Bus Selector : BusSelector  OutputSignals=World Position,qW2S,Body Velocity,Angular Rate
  Mux : Mux
  Quaternions to Rotation Angles : sharedtransform/Quaternions to Rotation Angles  rotationOrder=XYZ  aMode=aMode
      settings: SourceProductBaseCode=AE,PW,DR,MT,UV,VE
  Radians to Degrees : simulink_extras/Transformations/Radians to Degrees
  Radians to Degrees1 : simulink_extras/Transformations/Radians to Degrees
  states : Outport
  wires:
  Mux/1 -> states/1
  In1/1 -> Bus Selector/1
  Bus Selector/3 -> Mux/3  "<Body Velocity>"
  Bus Selector/1 -> Mux/1  "<World Position>"
  Bus Selector/4 -> Radians to Degrees/1  "<Angular Rate>"
  Radians to Degrees/1 -> Mux/4
  Quaternions to Rotation Angles/1 -> Radians to Degrees1/1
  Radians to Degrees1/1 -> Mux/2
  Bus Selector/2 -> Quaternions to Rotation Angles/1  "<qW2S>"

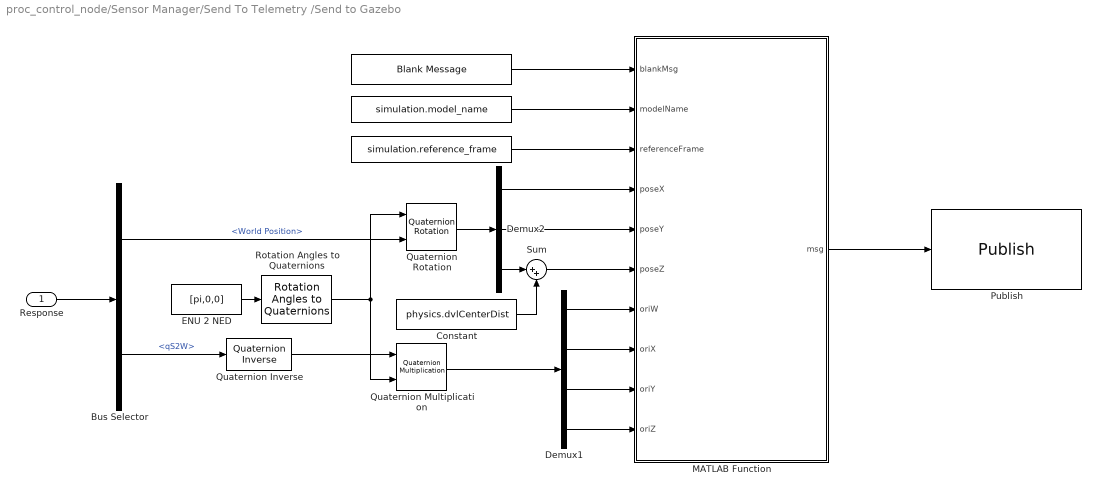
== system proc_control_node/Sensor Manager/Send To Telemetry /Send to Gazebo ==
  Response : Inport
  " " : Constant  Value=simulation.model_name  VectorParams1D=off
  "  " : Constant  Value=simulation.reference_frame
  "   " : robotlib/Blank Message  messageClass=Message  entityType=gazebo_msgs/ModelState  messageType=gazebo_msgs/ModelState  SampleTime=1/30  legacyBusStruct=off
  Bus Selector : BusSelector  OutputSignals=World Position,qS2W
  Constant : Constant  Value=physics.dvlCenterDist
  Demux1 : Demux
  Demux2 : Demux  Outputs=3
  ENU 2 NED : Constant  Value=[pi,0,0]
  MATLAB Function : MATLAB Function  TreatAsAtomicUnit=on  SystemSampleTime=1/30
  Publish : robotlib/Publish  topicSource=Select from ROS network  topic=/gazebo/set_model_state  messageType=gazebo_msgs/ModelState  legacyBusStruct=off  messageQueueLength=1
      link override SinkBlock: ROSTopic=/gazebo/set_model_state  ROSMessageType=gazebo_msgs/ModelState  SLBusName=SL_Bus_plant_gazebo_msgs_ModelState  ModelName=plant  BlockId=Pub_plant_206
  Quaternion Inverse : aerolibutil/Quaternion Inverse
  Quaternion Multiplication : aerolibutil/Quaternion Multiplication
  Quaternion Rotation : aerolibutil/Quaternion Rotation
  Rotation Angles to Quaternions : sharedtransform/Rotation Angles to Quaternions  rotationOrder=XYZ  aMode=aMode
      settings: SourceProductBaseCode=AE,PW,DR,MT,UV,VE
  Sum : Sum  Inputs=|++
  wires:
  "   "/1 -> MATLAB Function/1(blankMsg)
  "  "/1 -> MATLAB Function/3(referenceFrame)
  " "/1 -> MATLAB Function/2(modelName)
  Demux1/1 -> MATLAB Function/7(oriW)
  Demux1/2 -> MATLAB Function/8(oriX)
  Demux1/3 -> MATLAB Function/9(oriY)
  Demux1/4 -> MATLAB Function/10(oriZ)
  MATLAB Function/1(msg) -> Publish/1
  Response/1 -> Bus Selector/1
  Sum/1 -> MATLAB Function/6(poseZ)
  Constant/1 -> Sum/2
  Bus Selector/2 -> Quaternion Inverse/1  "<qS2W>"
  ENU 2 NED/1 -> Rotation Angles to Quaternions/1
  Rotation Angles to Quaternions/1 -> Quaternion Multiplication/2, Quaternion Rotation/1
  Bus Selector/1 -> Quaternion Rotation/2  "<World Position>"
  Demux2/3 -> Sum/1
  Demux2/2 -> MATLAB Function/5(poseY)
  Demux2/1 -> MATLAB Function/4(poseX)
  Quaternion Rotation/1 -> Demux2/1
  Quaternion Inverse/1 -> Quaternion Multiplication/1
  Quaternion Multiplication/1 -> Demux1/1

== system proc_control_node/Sensor Manager/Send To Telemetry /Send to Unity ==
  Response : Inport
  "   " : robotlib/Blank Message  messageClass=Message  entityType=geometry_msgs/Pose  messageType=geometry_msgs/Pose  SampleTime=1/60  legacyBusStruct=off
  Bus Selector : BusSelector  OutputSignals=World Position,qS2W
  Demux : Demux  Outputs=3
  MATLAB Function : MATLAB Function  TreatAsAtomicUnit=on  SystemSampleTime=1/60
  Publish : robotlib/Publish  topicSource=Specify your own  topic=/pos_rot  messageType=geometry_msgs/Pose  legacyBusStruct=off  messageQueueLength=1
      link override SinkBlock: ROSTopic=/gazebo/set_model_state  ROSMessageType=gazebo_msgs/ModelState  SLBusName=SL_Bus_plant_gazebo_msgs_ModelState  ModelName=plant  BlockId=Pub_plant_206
  Sum : Sum  Inputs=|++
  wires:
  Bus Selector/1 -> Demux/1  "<World Position>"
  "   "/1 -> MATLAB Function/1(blankMsg)
  MATLAB Function/1(msg) -> Publish/1
  Response/1 -> Bus Selector/1
  Sum/1 -> MATLAB Function/4(poseZ)
  Demux/1 -> MATLAB Function/2(poseX)
  Demux/2 -> MATLAB Function/3(poseY)
  Demux/3 -> Sum/1
  Bus Selector/2 -> MATLAB Function/5(quaternion)  "<qS2W>"

== system proc_control_node/Sensor Manager/Send Attitude To DVL/DVL2Ship/Subsystem2 ==
  Enable : EnablePort
  Rotation Angles to Quaternions : sharedtransform/Rotation Angles to Quaternions  rotationOrder=XYZ  aMode=aMode
      settings: SourceProductBaseCode=AE,PW,DR,MT,UV,VE
  si y devant : Constant  Value=[0,pi,-pi/2]
  Quat : Outport
  wires:
  si y devant/1 -> Rotation Angles to Quaternions/1
  Rotation Angles to Quaternions/1 -> Quat/1

== matlab function proc_control_node/Send Data to ROS/MATLAB Function3 ==
  data: blankMsg input; pwm input; msg output Bus: SL_Bus_proc_control_node_std_msgs_UInt16MultiArray
function msg = assignThrusterPwm(blankMsg, pwm)
msg = blankMsg;
msg.Data(1:8) = cast(pwm, 'uint16');
msg.Data_SL_Info.CurrentLength = uint32(8);

== matlab function proc_control_node/Sensor Manager/Send To Telemetry /Send to Gazebo/MATLAB Function ==
  data: blankMsg input; msg output Bus: SL_Bus_proc_control_node_gazebo_msgs_ModelState; modelName input; referenceFrame input; poseX input; poseY input; poseZ input; oriW input; oriX input; oriY input; oriZ input
function msg = assignGazeboModelStateInput(blankMsg, modelName, referenceFrame, poseX, poseY, poseZ, oriW, oriX, oriY, oriZ)
% assignStringInput - Assign a string in a ROS message to specified input string
%
% MSG = assignStringInput(blankMsg, STR) assigns the input string, STR, to
%  a string field in the ROS message, blankMsg, and outputs the updated
%  ROS message.
%
%  Inputs
%    blankMsg: A bus for a 'std_msgs/String' message. This is 
%        used to initialize the output.
%    str: An array of uint8 that will be assigned to the 'Data' field
%        in blankMsg. The entire array is assumed to be a valid sequence of
%        character ASCII values.
% 
%  Outputs:
%    msg: A bus for a 'std_msgs/String' message, with the 'Data'
%        field set to a string.

%   Copyright 2015 The MathWorks, Inc.
%#codegen

% Note: The datatype of 'msg' has been explicitly set to the appropriate 
% Simulink bus type ("Bus: SL_Bus_robotROSMessageUsageExample_std_msgs_String"). 
%
% If the model name is changed, the datatype needs to be changed as well:
%   1) Click "Edit Data" in the Editor toolstrip to open "Ports and Data Manager"
%   2) Select "msg". From the "Type" dropdown, select "--- Refresh data types ---"
%   3) Set datatype to "Bus: SL_Bus_<modelname>_std_msgs_String"
   
msg = blankMsg;

strLength = length(modelName);
msg.ModelName(1:strLength) = modelName;
msg.ModelName_SL_Info.CurrentLength = uint32(strLength);

strLength = length(referenceFrame);
msg.ReferenceFrame(1:strLength) = referenceFrame;
msg.ReferenceFrame_SL_Info.CurrentLength = uint32(strLength);

msg.Pose.Position.X = poseX;
msg.Pose.Position.Y = poseY;
msg.Pose.Position.Z = poseZ;

msg.Pose.Orientation.X = oriX;
msg.Pose.Orientation.Y = oriY;
msg.Pose.Orientation.Z = oriZ;
msg.Pose.Orientation.W = oriW;

== matlab function proc_control_node/Sensor Manager/Send DVL velocity To IMU/MATLAB Function1 ==
  data: blankMsg input; states input; msg output Bus: SL_Bus_proc_control_node_geometry_msgs_Twist
function msg = SendVelToIMU(blankMsg, states)
msg = blankMsg;


    
% Body velocity
    msg.Linear.X = states(1);
    msg.Linear.Y = states(2);
    msg.Linear.Z = states(3);

== matlab function proc_control_node/Send Data to ROS/Subsystem/MATLAB Function ==
  data: blankMsg input; targetReach input; mpcMode input; isMpcAlive input; msg output Bus: SL_Bus_proc_control_node_sonia_common_MpcInfo; tStatus input; mpcStatus input; OV input; MV input; MVR input; nx input; nu input
function msg = assignMpcInfo(blankMsg, targetReach, mpcMode, isMpcAlive, tStatus, mpcStatus, OV, MV, MVR, nx, nu )
   
msg = blankMsg;


msg.TargetReached = targetReach;
msg.IsMpcAlive = isMpcAlive;
msg.ThrustersStatus(1:nu) = tStatus;
msg.ThrustersStatus_SL_Info.CurrentLength = uint32(nu);

msg.MpcStatus = cast(mpcStatus,"int8");
msg.MpcMode = mpcMode;

msg.CurrentGains.OV(1:nx) = OV;
msg.CurrentGains.OV_SL_Info.CurrentLength = uint32(nx);

msg.CurrentGains.MV(1:nu) = MV;
msg.CurrentGains.MV_SL_Info.CurrentLength = uint32(nu);

msg.CurrentGains.MVR(1:nu) = MVR;
msg.CurrentGains.MVR_SL_Info.CurrentLength = uint32(nu);

== matlab function proc_control_node/Sensor Manager/Send Attitude To DVL/MATLAB Function1 ==
  data: blankMsg input; angles input; msg output Bus: SL_Bus_proc_control_node_geometry_msgs_Vector3
function msg = SendVelToIMU(blankMsg, angles)
msg = blankMsg;


    
% Body velocity
    msg.X = angles(1);
    msg.Y = angles(2);
    msg.Z = angles(3);

== matlab function proc_control_node/Send Data to ROS/MATLAB Function2 ==
  data: blankMsg input; pose input; msg output Bus: SL_Bus_proc_control_node_geometry_msgs_Pose
function msg = assigninitialWpts(blankMsg, pose)
msg = blankMsg;
msg.Position.X = pose(1);
msg.Position.Y = pose(2);
msg.Position.Z = pose(3);

msg.Orientation.W = pose(4);
msg.Orientation.X = pose(5);
msg.Orientation.Y = pose(6);
msg.Orientation.Z = pose(7);

== matlab function proc_control_node/Sensor Manager/Send To Telemetry /MATLAB Function1 ==
  data: blankMsg input; states input; msg output Bus: SL_Bus_proc_control_node_nav_msgs_Odometry
function msg = SendOdometry(blankMsg, states)
msg = blankMsg;

% World Position 
    msg.Pose.Pose.Position.X = states(1);
    msg.Pose.Pose.Position.Y = states(2);
    msg.Pose.Pose.Position.Z = states(3);
    
% Sub atitude
    msg.Pose.Pose.Orientation.X = states(4);
    msg.Pose.Pose.Orientation.Y = states(5);
    msg.Pose.Pose.Orientation.Z = states(6);
    
% Body velocity
    msg.Twist.Twist.Linear.X = states(7);
    msg.Twist.Twist.Linear.Y = states(8);
    msg.Twist.Twist.Linear.Z = states(9);
    
% Angular rates
    msg.Twist.Twist.Angular.X = states(10);
    msg.Twist.Twist.Angular.Y = states(11);
    msg.Twist.Twist.Angular.Z = states(12);

== matlab function proc_control_node/Sensor Manager/Send To Telemetry /Send to Unity/MATLAB Function ==
  data: blankMsg input; poseX input; poseY input; poseZ input; msg output Bus: SL_Bus_proc_control_node_geometry_msgs_Pose; quaternion input
function msg = assignUnityPoseRotInput(blankMsg, poseX, poseY, poseZ, quaternion)
% assignStringInput - Assign a string in a ROS message to specified input string
%
% MSG = assignStringInput(blankMsg, STR) assigns the input string, STR, to
%  a string field in the ROS message, blankMsg, and outputs the updated
%  ROS message.
%
%  Inputs
%    blankMsg: A bus for a 'std_msgs/String' message. This is 
%        used to initialize the output.
%    str: An array of uint8 that will be assigned to the 'Data' field
%        in blankMsg. The entire array is assumed to be a valid sequence of
%        character ASCII values.
% 
%  Outputs:
%    msg: A bus for a 'std_msgs/String' message, with the 'Data'
%        field set to a string.

%   Copyright 2015 The MathWorks, Inc.
%#codegen

% Note: The datatype of 'msg' has been explicitly set to the appropriate 
% Simulink bus type ("Bus: SL_Bus_robotROSMessageUsageExample_std_msgs_String"). 
%
% If the model name is changed, the datatype needs to be changed as well:
%   1) Click "Edit Data" in the Editor toolstrip to open "Ports and Data Manager"
%   2) Select "msg". From the "Type" dropdown, select "--- Refresh data types ---"
%   3) Set datatype to "Bus: SL_Bus_<modelname>_std_msgs_String"
   
msg = blankMsg;


msg.Position.X = poseX;
msg.Position.Y = poseY;
msg.Position.Z = poseZ;

msg.Orientation.X = quaternion(2);
msg.Orientation.Y = quaternion(3);
msg.Orientation.Z = quaternion(4);
msg.Orientation.W = quaternion(1);

== matlab function proc_control_node/Send Data to ROS/MATLAB Function1 ==
  data: blankMsg input; pwm input; msg output Bus: SL_Bus_proc_control_node_std_msgs_Int8MultiArray
function msg = assignThrusterNewton(blankMsg, pwm)
msg = blankMsg;
msg.Data(1:8) = cast(pwm, 'int8');
msg.Data_SL_Info.CurrentLength = uint32(8);

== matlab function proc_control_node/ROS Output/Send DVL msg/MATLAB Function ==
  data: blankMsg input; bodyVelocity input; msg output Bus: SL_Bus_proc_control_node_sonia_common_BodyVelocityDVL
function msg = DVLmessage(blankMsg, bodyVelocity)
% assignStringInput - Assign a string in a ROS message to specified input string
%
% MSG = assignStringInput(blankMsg, STR) assigns the input string, STR, to
%  a string field in the ROS message, blankMsg, and outputs the updated
%  ROS message.
%
%  Inputs
%    blankMsg: A bus for a 'std_msgs/String' message. This is 
%        used to initialize the output.
%    str: An array of uint8 that will be assigned to the 'Data' field
%        in blankMsg. The entire array is assumed to be a valid sequence of
%        character ASCII values.
% 
%  Outputs:
%    msg: A bus for a 'std_msgs/String' message, with the 'Data'
%        field set to a string.

%   Copyright 2015 The MathWorks, Inc.
%#codegen

% Note: The datatype of 'msg' has been explicitly set to the appropriate 
% Simulink bus type ("Bus: SL_Bus_robotROSMessageUsageExample_std_msgs_String"). 
%
% If the model name is changed, the datatype needs to be changed as well:
%   1) Click "Edit Data" in the Editor toolstrip to open "Ports and Data Manager"
%   2) Select "msg". From the "Type" dropdown, select "--- Refresh data types ---"
%   3) Set datatype to "Bus: SL_Bus_<modelname>_std_msgs_String"
   
msg = blankMsg;


msg.XVelBtm = bodyVelocity(1);
msg.YVelBtm = bodyVelocity(2);
msg.ZVelBtm = bodyVelocity(3);

== matlab function proc_control_node/ROS Output/Send IMU msg/MATLAB Function ==
  data: blankMsg input; angularRate input; quaternion input; msg output Bus: SL_Bus_proc_control_node_sensor_msgs_Imu; linearAcc input
function msg = IMUmessage(blankMsg, angularRate, quaternion, linearAcc)
% assignStringInput - Assign a string in a ROS message to specified input string
%
% MSG = assignStringInput(blankMsg, STR) assigns the input string, STR, to
%  a string field in the ROS message, blankMsg, and outputs the updated
%  ROS message.
%
%  Inputs
%    blankMsg: A bus for a 'std_msgs/String' message. This is 
%        used to initialize the output.
%    str: An array of uint8 that will be assigned to the 'Data' field
%        in blankMsg. The entire array is assumed to be a valid sequence of
%        character ASCII values.
% 
%  Outputs:
%    msg: A bus for a 'std_msgs/String' message, with the 'Data'
%        field set to a string.

%   Copyright 2015 The MathWorks, Inc.
%#codegen

% Note: The datatype of 'msg' has been explicitly set to the appropriate 
% Simulink bus type ("Bus: SL_Bus_robotROSMessageUsageExample_std_msgs_String"). 
%
% If the model name is changed, the datatype needs to be changed as well:
%   1) Click "Edit Data" in the Editor toolstrip to open "Ports and Data Manager"
%   2) Select "msg". From the "Type" dropdown, select "--- Refresh data types ---"
%   3) Set datatype to "Bus: SL_Bus_<modelname>_std_msgs_String"
   
msg = blankMsg;


msg.AngularVelocity.X = angularRate(1);
msg.AngularVelocity.Y = angularRate(2);
msg.AngularVelocity.Z = angularRate(3);

msg.Orientation.X = quaternion(2);
msg.Orientation.Y = quaternion(3);
msg.Orientation.Z = quaternion(4);
msg.Orientation.W = quaternion(1);

msg.LinearAcceleration.X = linearAcc(1);
msg.LinearAcceleration.Y = linearAcc(2);
msg.LinearAcceleration.Z = linearAcc(3);

== matlab function proc_control_node/ROS Output/Send to Gazebo/MATLAB Function ==
  data: blankMsg input; msg output Bus: SL_Bus_proc_control_node_gazebo_msgs_ModelState; modelName input; referenceFrame input; poseX input; poseY input; poseZ input; oriW input; oriX input; oriY input; oriZ input
function msg = assignGazeboModelStateInput(blankMsg, modelName, referenceFrame, poseX, poseY, poseZ, oriW, oriX, oriY, oriZ)
% assignStringInput - Assign a string in a ROS message to specified input string
%
% MSG = assignStringInput(blankMsg, STR) assigns the input string, STR, to
%  a string field in the ROS message, blankMsg, and outputs the updated
%  ROS message.
%
%  Inputs
%    blankMsg: A bus for a 'std_msgs/String' message. This is 
%        used to initialize the output.
%    str: An array of uint8 that will be assigned to the 'Data' field
%        in blankMsg. The entire array is assumed to be a valid sequence of
%        character ASCII values.
% 
%  Outputs:
%    msg: A bus for a 'std_msgs/String' message, with the 'Data'
%        field set to a string.

%   Copyright 2015 The MathWorks, Inc.
%#codegen

% Note: The datatype of 'msg' has been explicitly set to the appropriate 
% Simulink bus type ("Bus: SL_Bus_robotROSMessageUsageExample_std_msgs_String"). 
%
% If the model name is changed, the datatype needs to be changed as well:
%   1) Click "Edit Data" in the Editor toolstrip to open "Ports and Data Manager"
%   2) Select "msg". From the "Type" dropdown, select "--- Refresh data types ---"
%   3) Set datatype to "Bus: SL_Bus_<modelname>_std_msgs_String"
   
msg = blankMsg;

strLength = length(modelName);
msg.ModelName(1:strLength) = modelName;
msg.ModelName_SL_Info.CurrentLength = uint32(strLength);

strLength = length(referenceFrame);
msg.ReferenceFrame(1:strLength) = referenceFrame;
msg.ReferenceFrame_SL_Info.CurrentLength = uint32(strLength);

msg.Pose.Position.X = poseX;
msg.Pose.Position.Y = poseY;
msg.Pose.Position.Z = poseZ;

msg.Pose.Orientation.X = oriX;
msg.Pose.Orientation.Y = oriY;
msg.Pose.Orientation.Z = oriZ;
msg.Pose.Orientation.W = oriW;

== matlab function proc_control_node/ROS Output/Send to Unity/MATLAB Function ==
  data: blankMsg input; poseX input; poseY input; poseZ input; msg output Bus: SL_Bus_proc_control_node_geometry_msgs_Pose; quaternion input
function msg = assignUnityPoseRotInput(blankMsg, poseX, poseY, poseZ, quaternion)
   
msg = blankMsg;


msg.Position.X = poseX;
msg.Position.Y = poseY;
msg.Position.Z = poseZ;

msg.Orientation.X = quaternion(2);
msg.Orientation.Y = quaternion(3);
msg.Orientation.Z = quaternion(4);
msg.Orientation.W = quaternion(1);
